simulink library "TMCA_lib"  (Simulink 7.5)
settings: Solver=ode45  StartTime=0.0  StopTime=10.0  RelTol=1e-3
values from neighbouring files (symbols this model uses):
  pTMCA_A_BatCurrHi_C = Simulink.Parameter    [TMCA_par.m]
  pTMCA_A_BatCurrLo_C = Simulink.Parameter    [TMCA_par.m]
  pTMCA_bool_ACPtcConfig_C = Simulink.Parameter    [TMCA_par.m]
  pTMCA_bool_BatCoolACReqCtrl_C = Simulink.Parameter    [TMCA_par.m]
  pTMCA_bool_BatCoolACReqEnbl_C = Simulink.Parameter    [TMCA_par.m]
  pTMCA_bool_BatCoolEnbl_C = Simulink.Parameter    [TMCA_par.m]
  pTMCA_bool_BatHeatEnbl_C = Simulink.Parameter    [TMCA_par.m]
  pTMCA_bool_ChrgrValveCtrl_C = Simulink.Parameter    [TMCA_par.m]
  pTMCA_bool_ChrgrValveEnbl_C = Simulink.Parameter    [TMCA_par.m]
  pTMCA_bool_FanCtrlEnbl = Simulink.Parameter    [TMCA_par.m]
  pTMCA_bool_FanCtrlSwitch = Simulink.Parameter    [TMCA_par.m]
  pTMCA_bool_Mot1PmpEnbl_C = Simulink.Parameter    [TMCA_par.m]
  pTMCA_bool_Mot2PmpEnbl_C = Simulink.Parameter    [TMCA_par.m]
  pTMCA_bool_MotValveCtrl_C = Simulink.Parameter    [TMCA_par.m]
  pTMCA_bool_MotValveEnbl_C = Simulink.Parameter    [TMCA_par.m]
  pTMCA_bool_TMCoolEnbl_C = Simulink.Parameter    [TMCA_par.m]
  pTMCA_bool_WtrPmpCoolEnbl_C = Simulink.Parameter    [TMCA_par.m]
  pTMCA_bool_WtrPmpHeatEnbl_C = Simulink.Parameter    [TMCA_par.m]
  pTMCA_cnt_ACHeatTime_CUR = Simulink.Parameter    [TMCA_par.m]
  pTMCA_cnt_DCTempTime_CUR = Simulink.Parameter    [TMCA_par.m]
  pTMCA_cnt_TimeDwnLim_C = Simulink.Parameter    [TMCA_par.m]
  pTMCA_cnt_TimeUpLim_C = Simulink.Parameter    [TMCA_par.m]
  pTMCA_degC_AmbHiTempDisply_C = Simulink.Parameter    [TMCA_par.m]
  pTMCA_degC_BatCoolAmbHiTemp_C = Simulink.Parameter    [TMCA_par.m]
  pTMCA_degC_BatCoolAmbLoTemp_C = Simulink.Parameter    [TMCA_par.m]
  pTMCA_degC_BatCoolHiTemp_C = Simulink.Parameter    [TMCA_par.m]
  pTMCA_degC_BatCoolLoTemp_C = Simulink.Parameter    [TMCA_par.m]
  pTMCA_degC_BatHiTempDisply_C = Simulink.Parameter    [TMCA_par.m]
  pTMCA_degC_BatMaxT_CUR = Simulink.Parameter    [TMCA_par.m]
  pTMCA_degC_BatMaxTHiThd_C = Simulink.Parameter    [TMCA_par.m]
  pTMCA_degC_BatMaxTLoThd_C = Simulink.Parameter    [TMCA_par.m]
  pTMCA_degC_ChrgrHiTThd_C = Simulink.Parameter    [TMCA_par.m]
  pTMCA_degC_ChrgrLoTThd_C = Simulink.Parameter    [TMCA_par.m]
  pTMCA_degC_ChrgrTThd_CUR = Simulink.Parameter    [TMCA_par.m]
  pTMCA_degC_DcDcHiTThd_C = Simulink.Parameter    [TMCA_par.m]
  pTMCA_degC_DcDcLoTThd_C = Simulink.Parameter    [TMCA_par.m]
  pTMCA_degC_DcDcTThd_CUR = Simulink.Parameter    [TMCA_par.m]
  pTMCA_degC_MotWtrHiTThd_C = Simulink.Parameter    [TMCA_par.m]
  pTMCA_degC_MotWtrLoTThd_C = Simulink.Parameter    [TMCA_par.m]
  pTMCA_degC_MotWtrMaxTThd_C = Simulink.Parameter    [TMCA_par.m]
  pTMCA_degC_MotWtrMinTThd_C = Simulink.Parameter    [TMCA_par.m]
  pTMCA_pct_ACHeatPTCPWM_CUR = Simulink.Parameter    [TMCA_par.m]
  pTMCA_pct_BatWtrPmpPWM_CUR = Simulink.Parameter    [TMCA_par.m]
  pTMCA_pct_ChrgrWtrPmpPWM_CUR = Simulink.Parameter    [TMCA_par.m]
  pTMCA_pct_DcDcWtrPmpPWM_CUR = Simulink.Parameter    [TMCA_par.m]
  pTMCA_pct_DCHeatPTCPWM_CUR = Simulink.Parameter    [TMCA_par.m]
  pTMCA_pct_HeatPTCCtrl_C = Simulink.Parameter    [TMCA_par.m]
  pTMCA_pct_HeatPTCEnbl_C = Simulink.Parameter    [TMCA_par.m]
  pTMCA_pct_HeatrOffVal_C = Simulink.Parameter    [TMCA_par.m]
  pTMCA_pct_Mot1PmpPWMCtrl_C = Simulink.Parameter    [TMCA_par.m]
  pTMCA_pct_Mot2PmpPWMCtrl_C = Simulink.Parameter    [TMCA_par.m]
  pTMCA_pct_MotWtrPmpMaxSpd_C = Simulink.Parameter    [TMCA_par.m]
  pTMCA_pct_MotWtrPmpMinSpd_C = Simulink.Parameter    [TMCA_par.m]
  pTMCA_pct_MotWtrPmpNormSpd_C = Simulink.Parameter    [TMCA_par.m]
  pTMCA_pct_MotWtrPmpZeroSpd_C = Simulink.Parameter    [TMCA_par.m]
  pTMCA_pct_WtrPmpCoolCtrl_C = Simulink.Parameter    [TMCA_par.m]
  pTMCA_pct_WtrPmpHeatCtrl_C = Simulink.Parameter    [TMCA_par.m]
  pTMCA_s_ACDisChrgTimout_C = Simulink.Parameter    [TMCA_par.m]
  pTMCA_s_TFilSampleTi_C = Simulink.Parameter    [TMCA_par.m]
  pTMCA_st_AirCdnOn_C = Simulink.Parameter    [TMCA_par.m]
undefined symbols (not defined in the file or in its folder): AirCdnFanReqTyp, ChrgActStsTyp, MCUCoolReqTyp, p_bool_False_M, p_bool_True_M, PUDCoorrStsTyp
libraries: BaseOperationLib_Browser x197, PES_CZ_FAW x3, simulink x1
(part 1 of 2)
settings Model: Creator=wuaibin  LastModifiedBy=wuaibin

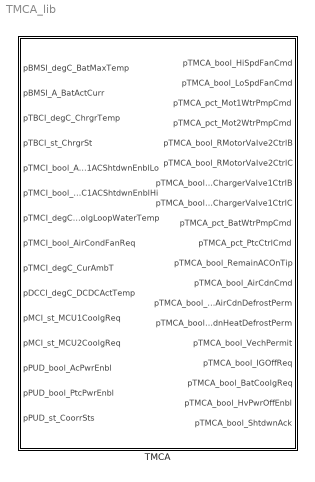
== system TMCA_lib ==
  TMCA : Subsystem  TreatAsAtomicUnit=on

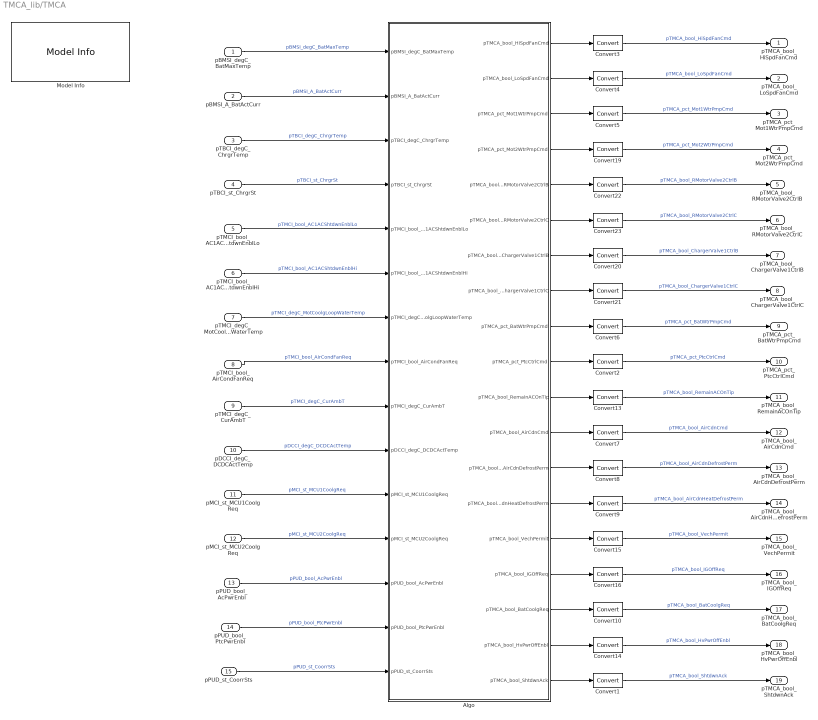
== system TMCA_lib/TMCA ==
  pBMSI_degC_BatMaxTemp : Inport  OutDataType=fixdt(1, 16)  OutScaling=2^0
  pBMSI_A_BatActCurr : Inport  Port=2  OutDataType=fixdt(1, 16)  OutScaling=2^0
  pTBCI_degC_ChrgrTemp : Inport  Port=3  OutDataType=fixdt(1, 16)  OutScaling=2^0
  pTBCI_st_ChrgrSt : Inport  Port=4  OutDataType=fixdt(1, 16)  OutScaling=2^0
  pTMCI_bool_AC1ACShtdwnEnblLo : Inport  Port=5  OutDataType=fixdt(1, 16)  OutScaling=2^0
  pTMCI_bool_AC1ACShtdwnEnblHi : Inport  Port=6  OutDataType=fixdt(1, 16)  OutScaling=2^0
  pTMCI_degC_MotCoolgLoopWaterTemp : Inport  Port=7  OutDataType=fixdt(1, 16)  OutScaling=2^0
  pTMCI_bool_AirCondFanReq : Inport  Port=8  OutDataType=fixdt(1, 16)  OutScaling=2^0
  pTMCI_degC_CurAmbT : Inport  Port=9  OutDataType=fixdt(1, 16)  OutScaling=2^0
  pDCCI_degC_DCDCActTemp : Inport  Port=10  OutDataType=fixdt(1, 16)  OutScaling=2^0
  pMCI_st_MCU1CoolgReq : Inport  Port=11  OutDataType=fixdt(1, 16)  OutScaling=2^0
  pMCI_st_MCU2CoolgReq : Inport  Port=12  OutDataType=fixdt(1, 16)  OutScaling=2^0
  pPUD_bool_AcPwrEnbl : Inport  Port=13
  pPUD_bool_PtcPwrEnbl : Inport  Port=14  OutDataType=fixdt(1, 16)  OutScaling=2^0
  pPUD_st_CoorrSts : Inport  Port=15
  Algo : Subsystem
  Convert{1..10,13..16,19..23} (19 alike) : DataTypeConversion  OutDataType=fixdt(1, 16)  OutScaling=2^0
  Model Info : simulink/Model-Wide Utilities/Model Info  SystemSampleTime=-1  InitialBlockCM=None  BlockCM=None  Frame=on  DisplayStringWithTags=Model Info\nCreated: %<Created>\nCreator: zhangqiang  HorizontalTextAlignment=Center  LeftAlignmentValue=0.5  SourceBlockDiagram=HQEV_HCU  TagMaxNumber=20
  pTMCA_bool_HiSpdFanCmd : Outport  OutDataType=fixdt(1, 16)  OutScaling=2^0
  pTMCA_bool_LoSpdFanCmd : Outport  Port=2  OutDataType=fixdt(1, 16)  OutScaling=2^0
  pTMCA_pct_Mot1WtrPmpCmd : Outport  Port=3  OutDataType=fixdt(1, 16)  OutScaling=2^0
  pTMCA_pct_Mot2WtrPmpCmd : Outport  Port=4  OutDataType=fixdt(1, 16)  OutScaling=2^0
  pTMCA_bool_RMotorValve2CtrlB : Outport  Port=5
  pTMCA_bool_RMotorValve2CtrlC : Outport  Port=6
  pTMCA_bool_ChargerValve1CtrlB : Outport  Port=7
  pTMCA_bool_ChargerValve1CtrlC : Outport  Port=8
  pTMCA_pct_BatWtrPmpCmd : Outport  Port=9  OutDataType=fixdt(1, 16)  OutScaling=2^0
  pTMCA_pct_PtcCtrlCmd : Outport  Port=10  OutDataType=fixdt(1, 16)  OutScaling=2^0
  pTMCA_bool_RemainACOnTip : Outport  Port=11  OutDataType=fixdt(1, 16)  OutScaling=2^0
  pTMCA_bool_AirCdnCmd : Outport  Port=12  OutDataType=fixdt(1, 16)  OutScaling=2^0
  pTMCA_bool_AirCdnDefrostPerm : Outport  Port=13  OutDataType=fixdt(1, 16)  OutScaling=2^0
  pTMCA_bool_AirCdnHeatDefrostPerm : Outport  Port=14  OutDataType=fixdt(1, 16)  OutScaling=2^0
  pTMCA_bool_VechPermit : Outport  Port=15  OutDataType=fixdt(1, 16)  OutScaling=2^0
  pTMCA_bool_IGOffReq : Outport  Port=16  OutDataType=fixdt(1, 16)  OutScaling=2^0
  pTMCA_bool_BatCoolgReq : Outport  Port=17  OutDataType=fixdt(1, 16)  OutScaling=2^0
  pTMCA_bool_HvPwrOffEnbl : Outport  Port=18  OutDataType=fixdt(1, 16)  OutScaling=2^0
  pTMCA_bool_ShtdwnAck : Outport  Port=19  OutDataType=fixdt(1, 16)  OutScaling=2^0
  wires:
  Convert2/1 -> pTMCA_pct_PtcCtrlCmd/1  "pTMCA_pct_PtcCtrlCmd"
  Convert5/1 -> pTMCA_pct_Mot1WtrPmpCmd/1  "pTMCA_pct_Mot1WtrPmpCmd"
  Convert6/1 -> pTMCA_pct_BatWtrPmpCmd/1  "pTMCA_pct_BatWtrPmpCmd"
  Convert10/1 -> pTMCA_bool_BatCoolgReq/1  "pTMCA_bool_BatCoolgReq"
  Convert19/1 -> pTMCA_pct_Mot2WtrPmpCmd/1  "pTMCA_pct_Mot2WtrPmpCmd"
  Convert13/1 -> pTMCA_bool_RemainACOnTip/1  "pTMCA_bool_RemainACOnTip"
  pPUD_st_CoorrSts/1 -> Algo/15(pPUD_st_CoorrSts)  "pPUD_st_CoorrSts"
  pPUD_bool_PtcPwrEnbl/1 -> Algo/14(pPUD_bool_PtcPwrEnbl)  "pPUD_bool_PtcPwrEnbl"
  pTMCI_degC_MotCoolgLoopWaterTemp/1 -> Algo/7(pTMCI_degC_MotCoolgLoopWaterTemp)  "pTMCI_degC_MotCoolgLoopWaterTemp"
  pTMCI_bool_AirCondFanReq/1 -> Algo/8(pTMCI_bool_AirCondFanReq)  "pTMCI_bool_AirCondFanReq"
  pTBCI_st_ChrgrSt/1 -> Algo/4(pTBCI_st_ChrgrSt)  "pTBCI_st_ChrgrSt"
  pTBCI_degC_ChrgrTemp/1 -> Algo/3(pTBCI_degC_ChrgrTemp)  "pTBCI_degC_ChrgrTemp"
  pDCCI_degC_DCDCActTemp/1 -> Algo/10(pDCCI_degC_DCDCActTemp)  "pDCCI_degC_DCDCActTemp"
  pMCI_st_MCU1CoolgReq/1 -> Algo/11(pMCI_st_MCU1CoolgReq)  "pMCI_st_MCU1CoolgReq"
  pMCI_st_MCU2CoolgReq/1 -> Algo/12(pMCI_st_MCU2CoolgReq)  "pMCI_st_MCU2CoolgReq"
  pBMSI_degC_BatMaxTemp/1 -> Algo/1(pBMSI_degC_BatMaxTemp)  "pBMSI_degC_BatMaxTemp"
  pTMCI_degC_CurAmbT/1 -> Algo/9(pTMCI_degC_CurAmbT)  "pTMCI_degC_CurAmbT"
  pPUD_bool_AcPwrEnbl/1 -> Algo/13(pPUD_bool_AcPwrEnbl)  "pPUD_bool_AcPwrEnbl"
  pBMSI_A_BatActCurr/1 -> Algo/2(pBMSI_A_BatActCurr)  "pBMSI_A_BatActCurr"
  pTMCI_bool_AC1ACShtdwnEnblLo/1 -> Algo/5(pTMCI_bool_AC1ACShtdwnEnblLo)  "pTMCI_bool_AC1ACShtdwnEnblLo"
  pTMCI_bool_AC1ACShtdwnEnblHi/1 -> Algo/6(pTMCI_bool_AC1ACShtdwnEnblHi)  "pTMCI_bool_AC1ACShtdwnEnblHi"
  Algo/1(pTMCA_bool_HiSpdFanCmd) -> Convert3/1
  Algo/2(pTMCA_bool_LoSpdFanCmd) -> Convert4/1
  Algo/3(pTMCA_pct_Mot1WtrPmpCmd) -> Convert5/1
  Algo/4(pTMCA_pct_Mot2WtrPmpCmd) -> Convert19/1
  Algo/5(pTMCA_bool_RMotorValve2CtrlB) -> Convert22/1
  Algo/6(pTMCA_bool_RMotorValve2CtrlC) -> Convert23/1
  Algo/7(pTMCA_bool_ChargerValve1CtrlB) -> Convert20/1
  Algo/8(pTMCA_bool_ChargerValve1CtrlC) -> Convert21/1
  Algo/9(pTMCA_pct_BatWtrPmpCmd) -> Convert6/1
  Algo/10(pTMCA_pct_PtcCtrlCmd) -> Convert2/1
  Algo/11(pTMCA_bool_RemainACOnTip) -> Convert13/1
  Algo/12(pTMCA_bool_AirCdnCmd) -> Convert7/1
  Algo/13(pTMCA_bool_AirCdnDefrostPerm) -> Convert8/1
  Algo/14(pTMCA_bool_AirCdnHeatDefrostPerm) -> Convert9/1
  Algo/15(pTMCA_bool_VechPermit) -> Convert15/1
  Algo/16(pTMCA_bool_IGOffReq) -> Convert16/1
  Algo/17(pTMCA_bool_BatCoolgReq) -> Convert10/1
  Algo/18(pTMCA_bool_HvPwrOffEnbl) -> Convert14/1
  Convert3/1 -> pTMCA_bool_HiSpdFanCmd/1  "pTMCA_bool_HiSpdFanCmd"
  Convert4/1 -> pTMCA_bool_LoSpdFanCmd/1  "pTMCA_bool_LoSpdFanCmd"
  Convert22/1 -> pTMCA_bool_RMotorValve2CtrlB/1  "pTMCA_bool_RMotorValve2CtrlB"
  Convert23/1 -> pTMCA_bool_RMotorValve2CtrlC/1  "pTMCA_bool_RMotorValve2CtrlC"
  Convert20/1 -> pTMCA_bool_ChargerValve1CtrlB/1  "pTMCA_bool_ChargerValve1CtrlB"
  Convert21/1 -> pTMCA_bool_ChargerValve1CtrlC/1  "pTMCA_bool_ChargerValve1CtrlC"
  Convert7/1 -> pTMCA_bool_AirCdnCmd/1  "pTMCA_bool_AirCdnCmd"
  Convert8/1 -> pTMCA_bool_AirCdnDefrostPerm/1  "pTMCA_bool_AirCdnDefrostPerm"
  Convert9/1 -> pTMCA_bool_AirCdnHeatDefrostPerm/1  "pTMCA_bool_AirCdnHeatDefrostPerm"
  Convert15/1 -> pTMCA_bool_VechPermit/1  "pTMCA_bool_VechPermit"
  Convert16/1 -> pTMCA_bool_IGOffReq/1  "pTMCA_bool_IGOffReq"
  Convert1/1 -> pTMCA_bool_ShtdwnAck/1  "pTMCA_bool_ShtdwnAck"
  Convert14/1 -> pTMCA_bool_HvPwrOffEnbl/1  "pTMCA_bool_HvPwrOffEnbl"
  Algo/19(pTMCA_bool_ShtdwnAck) -> Convert1/1

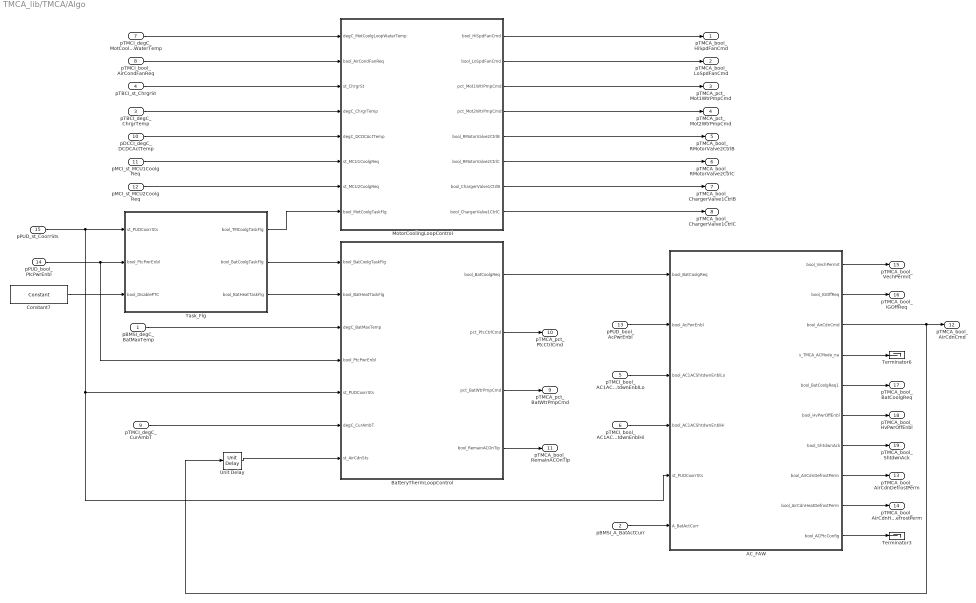
== system TMCA_lib/TMCA/Algo ==
  pBMSI_degC_BatMaxTemp : Inport  OutDataType=fixdt(1, 16)  OutScaling=2^0
  pBMSI_A_BatActCurr : Inport  Port=2  OutDataType=fixdt(1, 16)  OutScaling=2^0
  pTBCI_degC_ChrgrTemp : Inport  Port=3  OutDataType=fixdt(1, 16)  OutScaling=2^0
  pTBCI_st_ChrgrSt : Inport  Port=4  OutDataType=fixdt(1, 16)  OutScaling=2^0
  pTMCI_bool_AC1ACShtdwnEnblLo : Inport  Port=5  OutDataType=fixdt(1, 16)  OutScaling=2^0
  pTMCI_bool_AC1ACShtdwnEnblHi : Inport  Port=6  OutDataType=fixdt(1, 16)  OutScaling=2^0
  pTMCI_degC_MotCoolgLoopWaterTemp : Inport  Port=7  OutDataType=fixdt(1, 16)  OutScaling=2^0
  pTMCI_bool_AirCondFanReq : Inport  Port=8  OutDataType=fixdt(1, 16)  OutScaling=2^0
  pTMCI_degC_CurAmbT : Inport  Port=9  OutDataType=fixdt(1, 16)  OutScaling=2^0
  pDCCI_degC_DCDCActTemp : Inport  Port=10  OutDataType=fixdt(1, 16)  OutScaling=2^0
  pMCI_st_MCU1CoolgReq : Inport  Port=11  OutDataType=fixdt(1, 16)  OutScaling=2^0
  pMCI_st_MCU2CoolgReq : Inport  Port=12  OutDataType=fixdt(1, 16)  OutScaling=2^0
  pPUD_bool_AcPwrEnbl : Inport  Port=13  OutDataType=fixdt(1, 16)  OutScaling=2^0
  pPUD_bool_PtcPwrEnbl : Inport  Port=14
  pPUD_st_CoorrSts : Inport  Port=15  OutDataType=fixdt(1, 16)  OutScaling=2^0
  AC_FAW : Subsystem
  BatteryThermLoopControl : Subsystem
  Constant7 : BaseOperationLib_Browser/Sources&Sinks/Constant  Value=p_bool_False_M  OutMin=[]  OutMax=[]  OutDataType=fixdt(1, 16)  ConRadixGroup=Use specified scaling  OutScaling=2^0  OutDataTypeStr=Inherit: Inherit from 'Constant value'
  MotorCoolingLoopControl : Subsystem
  Task_Flg : Subsystem
  Terminator3 : Terminator
  Terminator6 : Terminator
  Unit Delay : BaseOperationLib_Browser/Discrete Unchanged /Unit Delay  X0=0  SampleTime=-1
  pTMCA_bool_HiSpdFanCmd : Outport  OutDataType=fixdt(1, 16)  OutScaling=2^0
  pTMCA_bool_LoSpdFanCmd : Outport  Port=2  OutDataType=fixdt(1, 16)  OutScaling=2^0
  pTMCA_pct_Mot1WtrPmpCmd : Outport  Port=3  OutDataType=fixdt(1, 16)  OutScaling=2^0
  pTMCA_pct_Mot2WtrPmpCmd : Outport  Port=4  PortDimensions=1  OutDataType=fixdt(1, 16)  OutScaling=2^0
  pTMCA_bool_RMotorValve2CtrlB : Outport  Port=5
  pTMCA_bool_RMotorValve2CtrlC : Outport  Port=6
  pTMCA_bool_ChargerValve1CtrlB : Outport  Port=7
  pTMCA_bool_ChargerValve1CtrlC : Outport  Port=8
  pTMCA_pct_BatWtrPmpCmd : Outport  Port=9  OutDataType=fixdt(1, 16)  OutScaling=2^0
  pTMCA_pct_PtcCtrlCmd : Outport  Port=10  OutDataType=fixdt(1, 16)  OutScaling=2^0
  pTMCA_bool_RemainACOnTip : Outport  Port=11  OutDataType=fixdt(1, 16)  OutScaling=2^0
  pTMCA_bool_AirCdnCmd : Outport  Port=12  OutDataType=fixdt(1, 16)  OutScaling=2^0
  pTMCA_bool_AirCdnDefrostPerm : Outport  Port=13  OutDataType=fixdt(1, 16)  OutScaling=2^0
  pTMCA_bool_AirCdnHeatDefrostPerm : Outport  Port=14  OutDataType=fixdt(1, 16)  OutScaling=2^0
  pTMCA_bool_VechPermit : Outport  Port=15  OutDataType=fixdt(1, 16)  OutScaling=2^0
  pTMCA_bool_IGOffReq : Outport  Port=16  OutDataType=fixdt(1, 16)  OutScaling=2^0
  pTMCA_bool_BatCoolgReq : Outport  Port=17  OutDataType=fixdt(1, 16)  OutScaling=2^0
  pTMCA_bool_HvPwrOffEnbl : Outport  Port=18  OutDataType=fixdt(1, 16)  OutScaling=2^0
  pTMCA_bool_ShtdwnAck : Outport  Port=19  OutDataType=fixdt(1, 16)  OutScaling=2^0
  wires:
  AC_FAW/3(bool_AirCdnCmd) -> pTMCA_bool_AirCdnCmd/1, Unit Delay/1
  Unit Delay/1 -> BatteryThermLoopControl/7(st_AirCdnSts)
  pTMCI_bool_AC1ACShtdwnEnblLo/1 -> AC_FAW/3(bool_AC1ACShtdwnEnblLo)
  AC_FAW/5(bool_BatCoolgReq1) -> pTMCA_bool_BatCoolgReq/1
  AC_FAW/4(s_TMCA_ACMode_na) -> Terminator6/1
  AC_FAW/8(bool_AirCdnDefrostPerm) -> pTMCA_bool_AirCdnDefrostPerm/1
  AC_FAW/9(bool_AirCdnHeatDefrostPerm) -> pTMCA_bool_AirCdnHeatDefrostPerm/1
  pTMCI_degC_MotCoolgLoopWaterTemp/1 -> MotorCoolingLoopControl/1(degC_MotCoolgLoopWaterTemp)
  pTMCI_bool_AirCondFanReq/1 -> MotorCoolingLoopControl/2(bool_AirCondFanReq)
  MotorCoolingLoopControl/2(bool_LoSpdFanCmd) -> pTMCA_bool_LoSpdFanCmd/1
  MotorCoolingLoopControl/1(bool_HiSpdFanCmd) -> pTMCA_bool_HiSpdFanCmd/1
  AC_FAW/10(bool_ACPtcConfig) -> Terminator3/1
  AC_FAW/1(bool_VechPermit) -> pTMCA_bool_VechPermit/1
  AC_FAW/2(bool_IGOffReq) -> pTMCA_bool_IGOffReq/1
  pTMCI_degC_CurAmbT/1 -> BatteryThermLoopControl/6(degC_CurAmbT)
  pTBCI_degC_ChrgrTemp/1 -> MotorCoolingLoopControl/4(degC_ChrgrTemp)
  pDCCI_degC_DCDCActTemp/1 -> MotorCoolingLoopControl/5(degC_DCDCActTemp)
  pMCI_st_MCU1CoolgReq/1 -> MotorCoolingLoopControl/6(st_MCU1CoolgReq)
  pMCI_st_MCU2CoolgReq/1 -> MotorCoolingLoopControl/7(st_MCU2CoolgReq)
  MotorCoolingLoopControl/3(pct_Mot1WtrPmpCmd) -> pTMCA_pct_Mot1WtrPmpCmd/1
  pBMSI_degC_BatMaxTemp/1 -> BatteryThermLoopControl/3(degC_BatMaxTemp)
  BatteryThermLoopControl/3(pct_BatWtrPmpCmd) -> pTMCA_pct_BatWtrPmpCmd/1
  BatteryThermLoopControl/1(bool_BatCoolgReq) -> AC_FAW/1(bool_BatCoolgReq)
  pPUD_bool_AcPwrEnbl/1 -> AC_FAW/2(bool_AcPwrEnbl)
  MotorCoolingLoopControl/4(pct_Mot2WtrPmpCmd) -> pTMCA_pct_Mot2WtrPmpCmd/1
  pTBCI_st_ChrgrSt/1 -> MotorCoolingLoopControl/3(st_ChrgrSt)
  MotorCoolingLoopControl/7(bool_ChargerValve1CtrlB) -> pTMCA_bool_ChargerValve1CtrlB/1
  MotorCoolingLoopControl/8(bool_ChargerValve1CtrlC) -> pTMCA_bool_ChargerValve1CtrlC/1
  MotorCoolingLoopControl/5(bool_RMotorValve2CtrlB) -> pTMCA_bool_RMotorValve2CtrlB/1
  MotorCoolingLoopControl/6(bool_RMotorValve2CtrlC) -> pTMCA_bool_RMotorValve2CtrlC/1
  BatteryThermLoopControl/4(bool_RemainACOnTip) -> pTMCA_bool_RemainACOnTip/1
  AC_FAW/6(bool_HvPwrOffEnbl) -> pTMCA_bool_HvPwrOffEnbl/1
  pPUD_bool_PtcPwrEnbl/1 -> BatteryThermLoopControl/4(bool_PtcPwrEnbl), Task_Flg/2(bool_PtcPwrEnbl)
  Constant7/1 -> Task_Flg/3(bool_DisablePTC)
  AC_FAW/7(bool_ShtdwnAck) -> pTMCA_bool_ShtdwnAck/1
  BatteryThermLoopControl/2(pct_PtcCtrlCmd) -> pTMCA_pct_PtcCtrlCmd/1
  Task_Flg/1(bool_TMCoolgTaskFlg) -> MotorCoolingLoopControl/8(bool_MotCoolgTaskFlg)
  Task_Flg/2(bool_BatCoolgTaskFlg) -> BatteryThermLoopControl/1(bool_BatCoolgTaskFlg)
  Task_Flg/3(bool_BatHeatTaskFlg) -> BatteryThermLoopControl/2(bool_BatHeatTaskFlg)
  pPUD_st_CoorrSts/1 -> Task_Flg/1(st_PUDCoorrSts), BatteryThermLoopControl/5(st_PUDCoorrSts), AC_FAW/5(st_PUDCoorrSts)
  pTMCI_bool_AC1ACShtdwnEnblHi/1 -> AC_FAW/4(bool_AC1ACShtdwnEnblHi)
  pBMSI_A_BatActCurr/1 -> AC_FAW/6(A_BatActCurr)

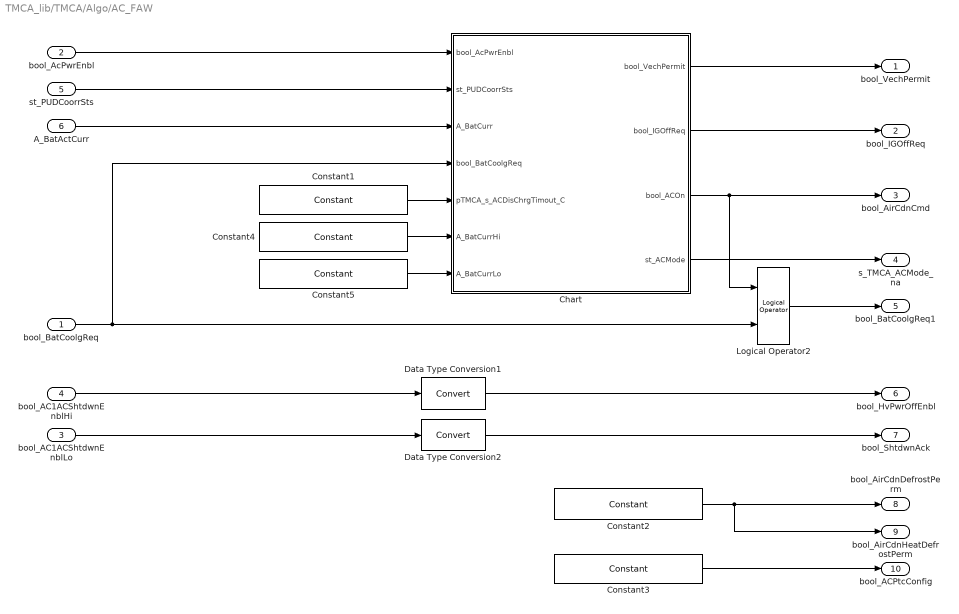
== system TMCA_lib/TMCA/Algo/AC_FAW ==
  bool_BatCoolgReq : Inport  OutDataType=fixdt(1, 16)  OutScaling=2^0
  bool_AcPwrEnbl : Inport  Port=2  OutDataType=fixdt(1, 16)  OutScaling=2^0
  bool_AC1ACShtdwnEnblLo : Inport  Port=3  OutDataType=fixdt(1, 16)  OutScaling=2^0
  bool_AC1ACShtdwnEnblHi : Inport  Port=4  OutDataType=fixdt(1, 16)  OutScaling=2^0
  st_PUDCoorrSts : Inport  Port=5  OutDataType=fixdt(1, 16)  OutScaling=2^0
  A_BatActCurr : Inport  Port=6  OutDataType=fixdt(1, 16)  OutScaling=2^0
  Chart : Stateflow chart  TreatAsAtomicUnit=on
  Constant1 : BaseOperationLib_Browser/Sources&Sinks/Constant  Value=pTMCA_s_ACDisChrgTimout_C  OutMin=[]  OutMax=[]  OutDataType=fixdt(1, 16)  ConRadixGroup=Use specified scaling  OutScaling=2^0  OutDataTypeStr=Inherit: Inherit from 'Constant value'
  Constant2 : BaseOperationLib_Browser/Sources&Sinks/Constant  Value=p_bool_False_M  OutMin=[]  OutMax=[]  OutDataType=fixdt(1, 16)  ConRadixGroup=Use specified scaling  OutScaling=2^0  OutDataTypeStr=Inherit: Inherit from 'Constant value'
  Constant3 : BaseOperationLib_Browser/Sources&Sinks/Constant  Value=pTMCA_bool_ACPtcConfig_C  OutMin=[]  OutMax=[]  OutDataType=fixdt(1, 16)  ConRadixGroup=Use specified scaling  OutScaling=2^0  OutDataTypeStr=Inherit: Inherit from 'Constant value'
  Constant4 : BaseOperationLib_Browser/Sources&Sinks/Constant  Value=pTMCA_A_BatCurrHi_C  OutMin=[]  OutMax=[]  OutDataType=fixdt(1, 16)  ConRadixGroup=Use specified scaling  OutScaling=2^0  OutDataTypeStr=Inherit: Inherit from 'Constant value'
  Constant5 : BaseOperationLib_Browser/Sources&Sinks/Constant  Value=pTMCA_A_BatCurrLo_C  OutMin=[]  OutMax=[]  OutDataType=fixdt(1, 16)  ConRadixGroup=Use specified scaling  OutScaling=2^0  OutDataTypeStr=Inherit: Inherit from 'Constant value'
  Data Type Conversion1 : DataTypeConversion  OutDataType=fixdt(1, 16)  OutScaling=2^0
  Data Type Conversion2 : DataTypeConversion  OutDataType=fixdt(1, 16)  OutScaling=2^0
  Logical Operator2 : BaseOperationLib_Browser/Logic Operations Changed/Logical Operator  Operator=AND  Inputs=2  AllPortsSameDT=on  OutDataTypeMode=Specify via dialog  LogicDataType=PDT_Bool  OutDataTypeStr=PDT_Bool
  bool_VechPermit : Outport  OutDataType=fixdt(1, 16)  OutScaling=2^0
  bool_IGOffReq : Outport  Port=2  OutDataType=fixdt(1, 16)  OutScaling=2^0
  bool_AirCdnCmd : Outport  Port=3  OutDataType=fixdt(1, 16)  OutScaling=2^0
  s_TMCA_ACMode_na : Outport  Port=4  PortDimensions=1  OutDataType=fixdt(1, 16)  OutScaling=2^0
  bool_BatCoolgReq1 : Outport  Port=5  OutDataType=fixdt(1, 16)  OutScaling=2^0
  bool_HvPwrOffEnbl : Outport  Port=6  PortDimensions=1  OutDataType=fixdt(1, 16)  OutScaling=2^0
  bool_ShtdwnAck : Outport  Port=7  OutDataType=fixdt(1, 16)  OutScaling=2^0
  bool_AirCdnDefrostPerm : Outport  Port=8  OutDataType=fixdt(1, 16)  OutScaling=2^0
  bool_AirCdnHeatDefrostPerm : Outport  Port=9  OutDataType=fixdt(1, 16)  OutScaling=2^0
  bool_ACPtcConfig : Outport  Port=10  OutDataType=fixdt(1, 16)  OutScaling=2^0
  wires:
  st_PUDCoorrSts/1 -> Chart/2(st_PUDCoorrSts)
  Logical Operator2/1 -> bool_BatCoolgReq1/1
  bool_BatCoolgReq/1 -> Logical Operator2/2, Chart/4(bool_BatCoolgReq)
  Chart/4(st_ACMode) -> s_TMCA_ACMode_na/1
  Chart/3(bool_ACOn) -> bool_AirCdnCmd/1, Logical Operator2/1
  Chart/2(bool_IGOffReq) -> bool_IGOffReq/1
  bool_AcPwrEnbl/1 -> Chart/1(bool_AcPwrEnbl)
  Chart/1(bool_VechPermit) -> bool_VechPermit/1
  Constant2/1 -> bool_AirCdnDefrostPerm/1, bool_AirCdnHeatDefrostPerm/1
  Constant3/1 -> bool_ACPtcConfig/1
  Data Type Conversion1/1 -> bool_HvPwrOffEnbl/1
  bool_AC1ACShtdwnEnblHi/1 -> Data Type Conversion1/1
  bool_AC1ACShtdwnEnblLo/1 -> Data Type Conversion2/1
  Data Type Conversion2/1 -> bool_ShtdwnAck/1
  A_BatActCurr/1 -> Chart/3(A_BatCurr)
  Constant1/1 -> Chart/5(pTMCA_s_ACDisChrgTimout_C)
  Constant4/1 -> Chart/6(A_BatCurrHi)
  Constant5/1 -> Chart/7(A_BatCurrLo)

== system TMCA_lib/TMCA/Algo/BatteryThermLoopControl ==
  bool_BatCoolgTaskFlg : Inport  OutDataType=fixdt(1, 16)  OutScaling=2^0
  bool_BatHeatTaskFlg : Inport  Port=2  OutDataType=fixdt(1, 16)  OutScaling=2^0
  degC_BatMaxTemp : Inport  Port=3  OutDataType=fixdt(1, 16)  OutScaling=2^0
  bool_PtcPwrEnbl : Inport  Port=4  OutDataType=fixdt(1, 16)  OutScaling=2^0
  st_PUDCoorrSts : Inport  Port=5  OutDataType=fixdt(1, 16)  OutScaling=2^0
  degC_CurAmbT : Inport  Port=6  OutDataType=fixdt(1, 16)  OutScaling=2^0
  st_AirCdnSts : Inport  Port=7  OutDataType=fixdt(1, 16)  OutScaling=2^0
  BatCoolingCtrl : Subsystem
  BatHeatingCtrl : Subsystem
  BatWaterPmpCtrl : Subsystem
  bool_BatCoolgReq : Outport  OutDataType=fixdt(1, 16)  OutScaling=2^0
  pct_PtcCtrlCmd : Outport  Port=2  OutDataType=fixdt(1, 16)  OutScaling=2^0
  pct_BatWtrPmpCmd : Outport  Port=3  OutDataType=fixdt(1, 16)  OutScaling=2^0
  bool_RemainACOnTip : Outport  Port=4  OutDataType=fixdt(1, 16)  OutScaling=2^0
  wires:
  bool_PtcPwrEnbl/1 -> BatHeatingCtrl/1(bool_PtcPwrEnbl)
  st_AirCdnSts/1 -> BatCoolingCtrl/3(st_AirCdnSts)
  degC_BatMaxTemp/1 -> BatCoolingCtrl/1(degC_BatMaxTemp), BatWaterPmpCtrl/3(degC_BatMaxTemp)
  BatHeatingCtrl/1(pct_PtcCtrlCmd) -> BatWaterPmpCtrl/2(pct_PtcCtrlCmd), pct_PtcCtrlCmd/1
  BatCoolingCtrl/1(bool_BatCoolgReq) -> BatWaterPmpCtrl/1(bool_BatCoolgReq), bool_BatCoolgReq/1
  BatWaterPmpCtrl/1(pct_BatWtrPmpCmd) -> pct_BatWtrPmpCmd/1
  BatCoolingCtrl/2(bool_RemainACOnTip) -> bool_RemainACOnTip/1
  degC_CurAmbT/1 -> BatCoolingCtrl/2(degC_CurAmbT)
  bool_BatCoolgTaskFlg/1 -> BatWaterPmpCtrl/4(bool_BatCoolgTaskFlg), BatCoolingCtrl/4(bool_BatCoolgTaskFlg)
  bool_BatHeatTaskFlg/1 -> BatHeatingCtrl/3(bool_BatHeatTaskFlg), BatWaterPmpCtrl/5(bool_BatHeatTaskFlg)
  st_PUDCoorrSts/1 -> BatHeatingCtrl/2(st_PUDCoorrSts)

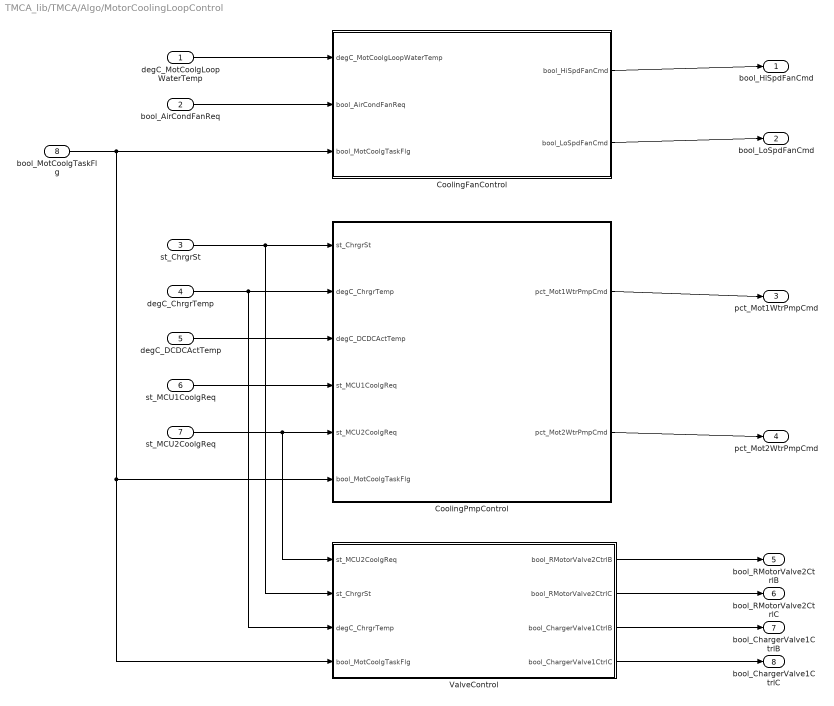
== system TMCA_lib/TMCA/Algo/MotorCoolingLoopControl ==
  degC_MotCoolgLoopWaterTemp : Inport  OutDataType=fixdt(1, 16)  OutScaling=2^0
  bool_AirCondFanReq : Inport  Port=2  OutDataType=fixdt(1, 16)  OutScaling=2^0
  st_ChrgrSt : Inport  Port=3  OutDataType=fixdt(1, 16)  OutScaling=2^0
  degC_ChrgrTemp : Inport  Port=4  OutDataType=fixdt(1, 16)  OutScaling=2^0
  degC_DCDCActTemp : Inport  Port=5  OutDataType=fixdt(1, 16)  OutScaling=2^0
  st_MCU1CoolgReq : Inport  Port=6  OutDataType=fixdt(1, 16)  OutScaling=2^0
  st_MCU2CoolgReq : Inport  Port=7  OutDataType=fixdt(1, 16)  OutScaling=2^0
  bool_MotCoolgTaskFlg : Inport  Port=8  OutDataType=fixdt(1, 16)  OutScaling=2^0
  CoolingFanControl : Subsystem
  CoolingPmpControl : Subsystem
  ValveControl : Subsystem
  bool_HiSpdFanCmd : Outport  OutDataType=fixdt(1, 16)  OutScaling=2^0
  bool_LoSpdFanCmd : Outport  Port=2  OutDataType=fixdt(1, 16)  OutScaling=2^0
  pct_Mot1WtrPmpCmd : Outport  Port=3  OutDataType=fixdt(1, 16)  OutScaling=2^0
  pct_Mot2WtrPmpCmd : Outport  Port=4  OutDataType=fixdt(1, 16)  OutScaling=2^0
  bool_RMotorValve2CtrlB : Outport  Port=5
  bool_RMotorValve2CtrlC : Outport  Port=6
  bool_ChargerValve1CtrlB : Outport  Port=7
  bool_ChargerValve1CtrlC : Outport  Port=8
  wires:
  CoolingFanControl/2(bool_LoSpdFanCmd) -> bool_LoSpdFanCmd/1
  CoolingFanControl/1(bool_HiSpdFanCmd) -> bool_HiSpdFanCmd/1
  bool_AirCondFanReq/1 -> CoolingFanControl/2(bool_AirCondFanReq)
  degC_MotCoolgLoopWaterTemp/1 -> CoolingFanControl/1(degC_MotCoolgLoopWaterTemp)
  CoolingPmpControl/1(pct_Mot1WtrPmpCmd) -> pct_Mot1WtrPmpCmd/1
  CoolingPmpControl/2(pct_Mot2WtrPmpCmd) -> pct_Mot2WtrPmpCmd/1
  st_MCU2CoolgReq/1 -> CoolingPmpControl/5(st_MCU2CoolgReq), ValveControl/1(st_MCU2CoolgReq)
  st_MCU1CoolgReq/1 -> CoolingPmpControl/4(st_MCU1CoolgReq)
  degC_DCDCActTemp/1 -> CoolingPmpControl/3(degC_DCDCActTemp)
  degC_ChrgrTemp/1 -> CoolingPmpControl/2(degC_ChrgrTemp), ValveControl/3(degC_ChrgrTemp)
  st_ChrgrSt/1 -> CoolingPmpControl/1(st_ChrgrSt), ValveControl/2(st_ChrgrSt)
  ValveControl/2(bool_RMotorValve2CtrlC) -> bool_RMotorValve2CtrlC/1
  ValveControl/1(bool_RMotorValve2CtrlB) -> bool_RMotorValve2CtrlB/1
  ValveControl/3(bool_ChargerValve1CtrlB) -> bool_ChargerValve1CtrlB/1
  ValveControl/4(bool_ChargerValve1CtrlC) -> bool_ChargerValve1CtrlC/1
  bool_MotCoolgTaskFlg/1 -> CoolingFanControl/3(bool_MotCoolgTaskFlg), CoolingPmpControl/6(bool_MotCoolgTaskFlg), ValveControl/4(bool_MotCoolgTaskFlg)

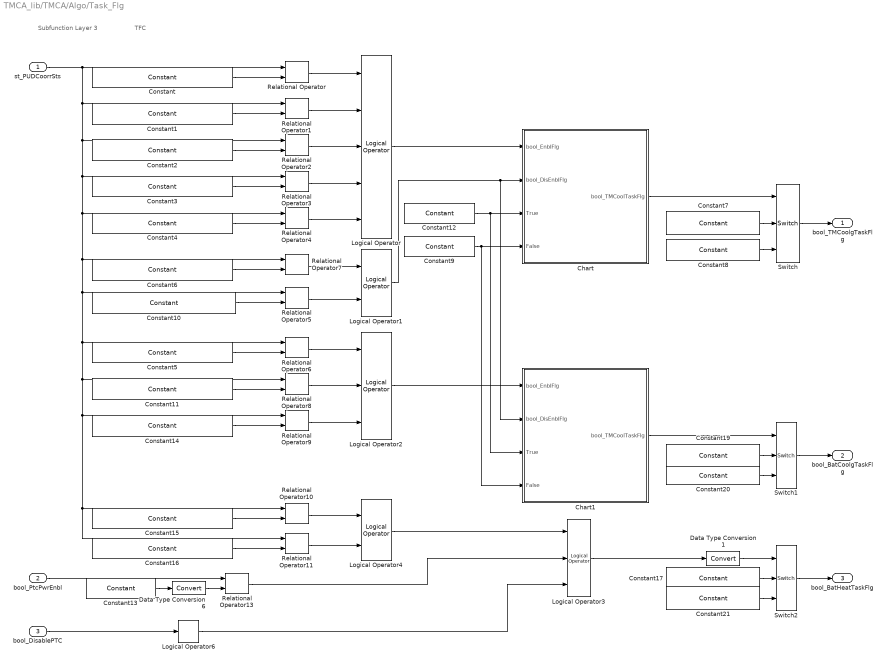
== system TMCA_lib/TMCA/Algo/Task_Flg ==
  note: TFC
  note: Subfunction Layer 3
  st_PUDCoorrSts : Inport
  bool_PtcPwrEnbl : Inport  Port=2
  bool_DisablePTC : Inport  Port=3
  Chart : Stateflow chart  TreatAsAtomicUnit=on
  Chart1 : Stateflow chart  TreatAsAtomicUnit=on
  Constant : BaseOperationLib_Browser/Sources&Sinks/Constant  Value=uint8(PUDCoorrStsTyp.PUD_DrvOn)  OutMin=[]  OutMax=[]  OutDataType=Enum: EgyCoorrStsTyp  ConRadixGroup=Best Precision: Vector-wise  OutScaling=[]  OutDataTypeStr=Inherit: Inherit from 'Constant value'
  Constant1 : BaseOperationLib_Browser/Sources&Sinks/Constant  Value=uint8(PUDCoorrStsTyp.PUD_ACChrgOn)  OutMin=[]  OutMax=[]  OutDataType=Enum: EgyCoorrStsTyp  ConRadixGroup=Best Precision: Vector-wise  OutScaling=[]  OutDataTypeStr=Inherit: Inherit from 'Constant value'
  Constant10 : BaseOperationLib_Browser/Sources&Sinks/Constant  Value=uint8(PUDCoorrStsTyp.PUD_EmgHVOFF_OK)  OutMin=[]  OutMax=[]  OutDataType=Enum: PtCoorrStsTyp  ConRadixGroup=Best Precision: Vector-wise  OutScaling=[]  OutDataTypeStr=Inherit: Inherit from 'Constant value'
  Constant11 : BaseOperationLib_Browser/Sources&Sinks/Constant  Value=uint8(PUDCoorrStsTyp.PUD_ACChrgOn)  OutMin=[]  OutMax=[]  OutDataType=Enum: EgyCoorrStsTyp  ConRadixGroup=Best Precision: Vector-wise  OutScaling=[]  OutDataTypeStr=Inherit: Inherit from 'Constant value'
  Constant12 : BaseOperationLib_Browser/Sources&Sinks/Constant  Value=p_bool_True_M  OutMin=[]  OutMax=[]  OutDataType=fixdt(1, 16)  ConRadixGroup=Use specified scaling  OutScaling=2^0  OutDataTypeStr=Inherit: Inherit from 'Constant value'
  Constant13 : BaseOperationLib_Browser/Sources&Sinks/Constant  Value=p_bool_True_M  OutMin=[]  OutMax=[]  OutDataType=fixdt(1, 16)  ConRadixGroup=Use specified scaling  OutScaling=2^0  OutDataTypeStr=Inherit: Inherit from 'Constant value'
  Constant14 : BaseOperationLib_Browser/Sources&Sinks/Constant  Value=uint8(PUDCoorrStsTyp.PUD_DCChrgOn)  OutMin=[]  OutMax=[]  OutDataType=Enum: EgyCoorrStsTyp  ConRadixGroup=Best Precision: Vector-wise  OutScaling=[]  OutDataTypeStr=Inherit: Inherit from 'Constant value'
  Constant15 : BaseOperationLib_Browser/Sources&Sinks/Constant  Value=uint8(PUDCoorrStsTyp.PUD_ACHeatOn)  OutMin=[]  OutMax=[]  OutDataType=Enum: EgyCoorrStsTyp  ConRadixGroup=Best Precision: Vector-wise  OutScaling=[]  OutDataTypeStr=Inherit: Inherit from 'Constant value'
  Constant16 : BaseOperationLib_Browser/Sources&Sinks/Constant  Value=uint8(PUDCoorrStsTyp.PUD_DCHeatOn)  OutMin=[]  OutMax=[]  OutDataType=Enum: EgyCoorrStsTyp  ConRadixGroup=Best Precision: Vector-wise  OutScaling=[]  OutDataTypeStr=Inherit: Inherit from 'Constant value'
  Constant17 : BaseOperationLib_Browser/Sources&Sinks/Constant  Value=pTMCA_bool_BatHeatEnbl_C  OutMin=[]  OutMax=[]  OutDataType=fixdt(1, 16)  ConRadixGroup=Use specified scaling  OutScaling=2^0  OutDataTypeStr=Inherit: Inherit from 'Constant value'
  Constant19 : BaseOperationLib_Browser/Sources&Sinks/Constant  Value=pTMCA_bool_BatCoolEnbl_C  OutMin=[]  OutMax=[]  OutDataType=fixdt(1, 16)  ConRadixGroup=Use specified scaling  OutScaling=2^0  OutDataTypeStr=Inherit: Inherit from 'Constant value'
  Constant2 : BaseOperationLib_Browser/Sources&Sinks/Constant  Value=uint8(PUDCoorrStsTyp.PUD_DCChrgOn)  OutMin=[]  OutMax=[]  OutDataType=Enum: EgyCoorrStsTyp  ConRadixGroup=Best Precision: Vector-wise  OutScaling=[]  OutDataTypeStr=Inherit: Inherit from 'Constant value'
  Constant{8..9,20..21} (4 alike) : BaseOperationLib_Browser/Sources&Sinks/Constant  Value=p_bool_False_M  OutMin=[]  OutMax=[]  OutDataType=fixdt(1, 16)  ConRadixGroup=Use specified scaling  OutScaling=2^0  OutDataTypeStr=Inherit: Inherit from 'Constant value'
  Constant3 : BaseOperationLib_Browser/Sources&Sinks/Constant  Value=uint8(PUDCoorrStsTyp.PUD_ACHeatOn)  OutMin=[]  OutMax=[]  OutDataType=Enum: EgyCoorrStsTyp  ConRadixGroup=Best Precision: Vector-wise  OutScaling=[]  OutDataTypeStr=Inherit: Inherit from 'Constant value'
  Constant4 : BaseOperationLib_Browser/Sources&Sinks/Constant  Value=uint8(PUDCoorrStsTyp.PUD_DCHeatOn)  OutMin=[]  OutMax=[]  OutDataType=Enum: EgyCoorrStsTyp  ConRadixGroup=Best Precision: Vector-wise  OutScaling=[]  OutDataTypeStr=Inherit: Inherit from 'Constant value'
  Constant5 : BaseOperationLib_Browser/Sources&Sinks/Constant  Value=uint8(PUDCoorrStsTyp.PUD_DrvOn)  OutMin=[]  OutMax=[]  OutDataType=Enum: EgyCoorrStsTyp  ConRadixGroup=Best Precision: Vector-wise  OutScaling=[]  OutDataTypeStr=Inherit: Inherit from 'Constant value'
  Constant6 : BaseOperationLib_Browser/Sources&Sinks/Constant  Value=uint8(PUDCoorrStsTyp.PUD_HVOFF_OK)  OutMin=[]  OutMax=[]  OutDataType=Enum: PtCoorrStsTyp  ConRadixGroup=Best Precision: Vector-wise  OutScaling=[]  OutDataTypeStr=Inherit: Inherit from 'Constant value'
  Constant7 : BaseOperationLib_Browser/Sources&Sinks/Constant  Value=pTMCA_bool_TMCoolEnbl_C  OutMin=[]  OutMax=[]  OutDataType=fixdt(1, 16)  ConRadixGroup=Use specified scaling  OutScaling=2^0  OutDataTypeStr=Inherit: Inherit from 'Constant value'
  Data Type Conversion1 : DataTypeConversion  OutDataType=fixdt(1, 16)  OutScaling=2^0
  Data Type Conversion6 : DataTypeConversion  OutDataType=fixdt(1, 16)  OutScaling=2^0
  Logical Operator : BaseOperationLib_Browser/Logic Operations Changed/Logical Operator  Operator=OR  Inputs=5  AllPortsSameDT=on  OutDataTypeMode=Specify via dialog  LogicDataType=PDT_Bool  OutDataTypeStr=PDT_Bool
  Logical Operator1 : BaseOperationLib_Browser/Logic Operations Changed/Logical Operator  Operator=OR  Inputs=2  AllPortsSameDT=on  OutDataTypeMode=Specify via dialog  LogicDataType=PDT_Bool  OutDataTypeStr=PDT_Bool
  Logical Operator2 : BaseOperationLib_Browser/Logic Operations Changed/Logical Operator  Operator=OR  Inputs=3  AllPortsSameDT=on  OutDataTypeMode=Specify via dialog  LogicDataType=PDT_Bool  OutDataTypeStr=PDT_Bool
  Logical Operator3 : BaseOperationLib_Browser/Logic Operations Changed/Logical Operator  Operator=AND  Inputs=3  AllPortsSameDT=on  OutDataTypeMode=Specify via dialog  LogicDataType=PDT_Bool  OutDataTypeStr=PDT_Bool
  Logical Operator4 : BaseOperationLib_Browser/Logic Operations Changed/Logical Operator  Operator=OR  Inputs=2  AllPortsSameDT=on  OutDataTypeMode=Specify via dialog  LogicDataType=PDT_Bool  OutDataTypeStr=PDT_Bool
  Logical Operator6 : BaseOperationLib_Browser/Logic Operations Changed/Logical Operator  Operator=NOT  Inputs=2  AllPortsSameDT=on  OutDataTypeMode=Specify via dialog  LogicDataType=PDT_Bool  OutDataTypeStr=PDT_Bool
  Relational Operator{,1..11,13} (13 alike) : BaseOperationLib_Browser/Logic Operations Changed/Relational Operator  Operator===  InputSameDT=on  LogicOutDataTypeMode=Specify via dialog  LogicDataType=PDT_Bool  OutDataTypeStr=PDT_Bool
  Switch : BaseOperationLib_Browser/Signal Routing Changed/Switch  Criteria=u2 ~= 0  Threshold=1  InputSameDT=on  OutMin=[]  OutMax=[]  OutDataType=fixdt(1,16,0)  OutScaling=[]  SaturateOnIntegerOverflow=on
  Switch1 : BaseOperationLib_Browser/Signal Routing Changed/Switch  Criteria=u2 ~= 0  Threshold=1  InputSameDT=on  OutMin=[]  OutMax=[]  OutDataType=fixdt(1,16,0)  OutScaling=[]  SaturateOnIntegerOverflow=on
  Switch2 : BaseOperationLib_Browser/Signal Routing Changed/Switch  Criteria=u2 ~= 0  Threshold=1  InputSameDT=on  OutMin=[]  OutMax=[]  OutDataType=fixdt(1,16,0)  OutScaling=[]  SaturateOnIntegerOverflow=on
  bool_TMCoolgTaskFlg : Outport  OutDataType=fixdt(1, 16)  OutScaling=2^0
  bool_BatCoolgTaskFlg : Outport  Port=2  OutDataType=fixdt(1, 16)  OutScaling=2^0
  bool_BatHeatTaskFlg : Outport  Port=3  OutDataType=fixdt(1, 16)  OutScaling=2^0
  wires:
  Constant1/1 -> Relational Operator1/2
  Constant2/1 -> Relational Operator2/2
  Constant3/1 -> Relational Operator3/2
  Relational Operator/1 -> Logical Operator/1
  Relational Operator1/1 -> Logical Operator/2
  Relational Operator2/1 -> Logical Operator/3
  Relational Operator3/1 -> Logical Operator/4
  Relational Operator4/1 -> Logical Operator/5
  st_PUDCoorrSts/1 -> Relational Operator/1, Relational Operator1/1, Relational Operator2/1, Relational Operator3/1, Relational Operator4/1, Relational Operator7/1, Relational Operator8/1, Relational Operator9/1, Relational Operator10/1, Relational Operator11/1, Relational Operator6/1, Relational Operator5/1
  Logical Operator/1 -> Chart/1(bool_EnblFlg)
  Constant9/1 -> Chart1/4(False), Chart/4(False)
  Constant12/1 -> Chart1/3(True), Chart/3(True)
  Constant6/1 -> Relational Operator7/2
  Logical Operator1/1 -> Chart1/2(bool_DisEnblFlg), Chart/2(bool_DisEnblFlg)
  Switch/1 -> bool_TMCoolgTaskFlg/1
  Constant7/1 -> Switch/2
  Chart/1(bool_TMCoolTaskFlg) -> Switch/1
  Constant10/1 -> Relational Operator5/2
  Relational Operator7/1 -> Logical Operator1/1
  Relational Operator5/1 -> Logical Operator1/2
  Constant/1 -> Relational Operator/2
  Constant4/1 -> Relational Operator4/2
  Constant8/1 -> Switch/3
  Data Type Conversion6/1 -> Relational Operator13/2
  Constant20/1 -> Switch1/3
  Constant19/1 -> Switch1/2
  Switch1/1 -> bool_BatCoolgTaskFlg/1
  Relational Operator11/1 -> Logical Operator4/2
  Relational Operator10/1 -> Logical Operator4/1
  Relational Operator9/1 -> Logical Operator2/3
  Relational Operator8/1 -> Logical Operator2/2
  Relational Operator6/1 -> Logical Operator2/1
  Constant16/1 -> Relational Operator11/2
  Constant15/1 -> Relational Operator10/2
  Constant14/1 -> Relational Operator9/2
  Constant11/1 -> Relational Operator8/2
  Constant5/1 -> Relational Operator6/2
  Constant17/1 -> Switch2/2
  Logical Operator4/1 -> Logical Operator3/1
  Switch2/1 -> bool_BatHeatTaskFlg/1
  Logical Operator3/1 -> Data Type Conversion1/1
  Constant21/1 -> Switch2/3
  bool_PtcPwrEnbl/1 -> Relational Operator13/1
  Constant13/1 -> Data Type Conversion6/1
  Relational Operator13/1 -> Logical Operator3/2
  Data Type Conversion1/1 -> Switch2/1
  Chart1/1(bool_TMCoolTaskFlg) -> Switch1/1
  bool_DisablePTC/1 -> Logical Operator6/1
  Logical Operator6/1 -> Logical Operator3/3
  Logical Operator2/1 -> Chart1/1(bool_EnblFlg)

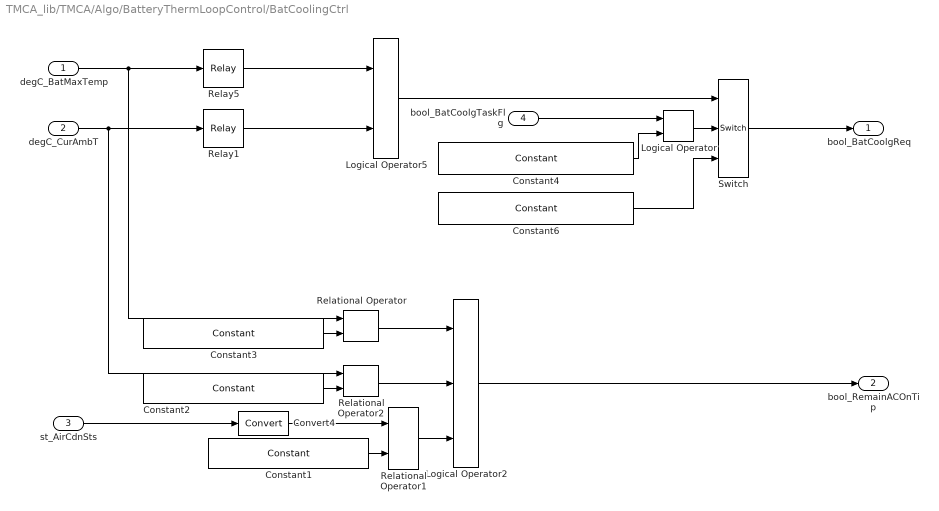
== system TMCA_lib/TMCA/Algo/BatteryThermLoopControl/BatCoolingCtrl ==
  degC_BatMaxTemp : Inport  OutDataType=fixdt(1, 16)  OutScaling=2^0
  degC_CurAmbT : Inport  Port=2  OutDataType=fixdt(1, 16)  OutScaling=2^0
  st_AirCdnSts : Inport  Port=3  OutDataType=fixdt(1, 16)  OutScaling=2^0
  bool_BatCoolgTaskFlg : Inport  Port=4  OutDataType=fixdt(1, 16)  OutScaling=2^0
  Constant1 : BaseOperationLib_Browser/Sources&Sinks/Constant  Value=pTMCA_st_AirCdnOn_C  OutMin=[]  OutMax=[]  OutDataType=fixdt(1, 16)  ConRadixGroup=Use specified scaling  OutScaling=2^0  OutDataTypeStr=Inherit: Inherit from 'Constant value'
  Constant2 : BaseOperationLib_Browser/Sources&Sinks/Constant  Value=pTMCA_degC_AmbHiTempDisply_C  OutMin=[]  OutMax=[]  OutDataType=fixdt(1, 16)  ConRadixGroup=Use specified scaling  OutScaling=2^0  OutDataTypeStr=Inherit: Inherit from 'Constant value'
  Constant3 : BaseOperationLib_Browser/Sources&Sinks/Constant  Value=pTMCA_degC_BatHiTempDisply_C  OutMin=[]  OutMax=[]  OutDataType=fixdt(1, 16)  ConRadixGroup=Use specified scaling  OutScaling=2^0  OutDataTypeStr=Inherit: Inherit from 'Constant value'
  Constant4 : BaseOperationLib_Browser/Sources&Sinks/Constant  Value=pTMCA_bool_BatCoolACReqEnbl_C  OutMin=[]  OutMax=[]  OutDataType=fixdt(1, 16)  ConRadixGroup=Use specified scaling  OutScaling=2^0  OutDataTypeStr=Inherit: Inherit from 'Constant value'
  Constant6 : BaseOperationLib_Browser/Sources&Sinks/Constant  Value=pTMCA_bool_BatCoolACReqCtrl_C  OutMin=[]  OutMax=[]  OutDataType=fixdt(1, 16)  ConRadixGroup=Use specified scaling  OutScaling=2^0  OutDataTypeStr=Inherit: Inherit from 'Constant value'
  Convert4 : DataTypeConversion  OutDataType=fixdt(1, 16)  OutScaling=2^0
  Logical Operator : BaseOperationLib_Browser/Logic Operations Changed/Logical Operator  Operator=AND  Inputs=2  AllPortsSameDT=on  OutDataTypeMode=Specify via dialog  LogicDataType=PDT_Bool  OutDataTypeStr=PDT_Bool
  Logical Operator2 : BaseOperationLib_Browser/Logic Operations Changed/Logical Operator  Operator=AND  Inputs=3  AllPortsSameDT=on  OutDataTypeMode=Specify via dialog  LogicDataType=PDT_Bool  OutDataTypeStr=PDT_Bool
  Logical Operator5 : BaseOperationLib_Browser/Logic Operations Changed/Logical Operator  Operator=AND  Inputs=2  AllPortsSameDT=on  OutDataTypeMode=Specify via dialog  LogicDataType=PDT_Bool  OutDataTypeStr=PDT_Bool
  Relational Operator : BaseOperationLib_Browser/Logic Operations Changed/Relational Operator  Operator=<=  InputSameDT=on  LogicOutDataTypeMode=Specify via dialog  LogicDataType=PDT_Bool  OutDataTypeStr=PDT_Bool
  Relational Operator1 : BaseOperationLib_Browser/Logic Operations Changed/Relational Operator  Operator===  InputSameDT=on  LogicOutDataTypeMode=Specify via dialog  LogicDataType=PDT_Bool  OutDataTypeStr=PDT_Bool
  Relational Operator2 : BaseOperationLib_Browser/Logic Operations Changed/Relational Operator  Operator=<=  InputSameDT=on  LogicOutDataTypeMode=Specify via dialog  LogicDataType=PDT_Bool  OutDataTypeStr=PDT_Bool
  Relay1 : BaseOperationLib_Browser/Discontinuities Changed/Relay  OnSwitchValue=pTMCA_degC_BatCoolAmbHiTemp_C  OffSwitchValue=pTMCA_degC_BatCoolAmbLoTemp_C  OnOutputValue=p_bool_True_M  OffOutputValue=p_bool_False_M  OutMin=[]  OutMax=[]  OutDataType=fixdt(1, 16)  ConRadixGroup=Use specified scaling  OutScaling=2^0  OutDataTypeStr=Inherit: Inherit via back propagation
      settings: AttributesFormatString=%<OnSwitchValue> OnOut %<OnOutputValue>\n%<OffSwitchValue> OffOut %<OffOutputValue>
  Relay5 : BaseOperationLib_Browser/Discontinuities Changed/Relay  OnSwitchValue=pTMCA_degC_BatCoolHiTemp_C  OffSwitchValue=pTMCA_degC_BatCoolLoTemp_C  OnOutputValue=p_bool_True_M  OffOutputValue=p_bool_False_M  OutMin=[]  OutMax=[]  OutDataType=fixdt(1, 16)  ConRadixGroup=Use specified scaling  OutScaling=2^0  OutDataTypeStr=Inherit: Inherit via back propagation
      settings: AttributesFormatString=%<OnSwitchValue> OnOut %<OnOutputValue>\n%<OffSwitchValue> OffOut %<OffOutputValue>
  Switch : BaseOperationLib_Browser/Signal Routing Changed/Switch  Criteria=u2 ~= 0  Threshold=1  InputSameDT=on  OutMin=[]  OutMax=[]  OutDataType=fixdt(1,16,0)  OutScaling=[]  SaturateOnIntegerOverflow=on
  bool_BatCoolgReq : Outport  OutDataType=fixdt(1, 16)  OutScaling=2^0
  bool_RemainACOnTip : Outport  Port=2  OutDataType=fixdt(1, 16)  OutScaling=2^0
  wires:
  Constant3/1 -> Relational Operator/2
  Constant2/1 -> Relational Operator2/2
  Relational Operator2/1 -> Logical Operator2/2
  Relational Operator/1 -> Logical Operator2/1
  Relational Operator1/1 -> Logical Operator2/3
  degC_CurAmbT/1 -> Relational Operator2/1, Relay1/1
  Relay1/1 -> Logical Operator5/2
  bool_BatCoolgTaskFlg/1 -> Logical Operator/1
  Constant4/1 -> Logical Operator/2
  Logical Operator/1 -> Switch/2
  Convert4/1 -> Relational Operator1/1
  Logical Operator2/1 -> bool_RemainACOnTip/1
  Logical Operator5/1 -> Switch/1
  st_AirCdnSts/1 -> Convert4/1
  Constant1/1 -> Relational Operator1/2
  degC_BatMaxTemp/1 -> Relational Operator/1, Relay5/1
  Relay5/1 -> Logical Operator5/1
  Constant6/1 -> Switch/3
  Switch/1 -> bool_BatCoolgReq/1

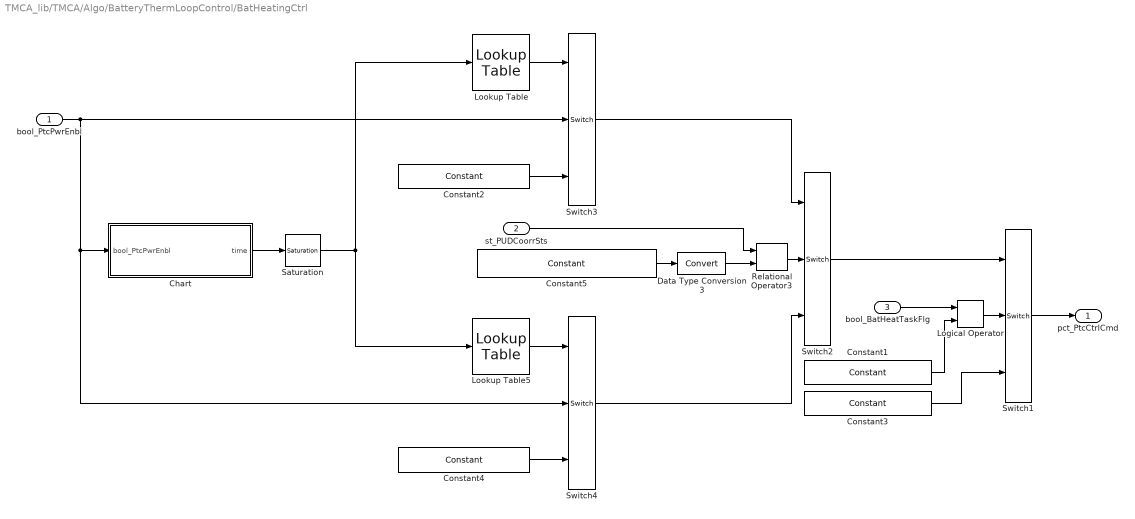
== system TMCA_lib/TMCA/Algo/BatteryThermLoopControl/BatHeatingCtrl ==
  bool_PtcPwrEnbl : Inport  OutDataType=fixdt(1, 16)  OutScaling=2^0
  st_PUDCoorrSts : Inport  Port=2  OutDataType=fixdt(1, 16)  OutScaling=2^0
  bool_BatHeatTaskFlg : Inport  Port=3  OutDataType=fixdt(1, 16)  OutScaling=2^0
  Chart : Stateflow chart  TreatAsAtomicUnit=on
  Constant1 : BaseOperationLib_Browser/Sources&Sinks/Constant  Value=pTMCA_pct_HeatPTCEnbl_C  OutMin=[]  OutMax=[]  OutDataType=fixdt(1, 16)  ConRadixGroup=Use specified scaling  OutScaling=2^0  OutDataTypeStr=Inherit: Inherit from 'Constant value'
  Constant2 : BaseOperationLib_Browser/Sources&Sinks/Constant  Value=pTMCA_pct_HeatrOffVal_C  OutMin=[]  OutMax=[]  OutDataType=fixdt(1, 16)  ConRadixGroup=Use specified scaling  OutScaling=2^0  OutDataTypeStr=Inherit: Inherit from 'Constant value'
  Constant3 : BaseOperationLib_Browser/Sources&Sinks/Constant  Value=pTMCA_pct_HeatPTCCtrl_C  OutMin=[]  OutMax=[]  OutDataType=fixdt(1, 16)  ConRadixGroup=Use specified scaling  OutScaling=2^0  OutDataTypeStr=Inherit: Inherit from 'Constant value'
  Constant4 : BaseOperationLib_Browser/Sources&Sinks/Constant  Value=pTMCA_pct_HeatrOffVal_C  OutMin=[]  OutMax=[]  OutDataType=fixdt(1, 16)  ConRadixGroup=Use specified scaling  OutScaling=2^0  OutDataTypeStr=Inherit: Inherit from 'Constant value'
  Constant5 : BaseOperationLib_Browser/Sources&Sinks/Constant  Value=uint8(PUDCoorrStsTyp.PUD_ACHeatOn)  OutMin=[]  OutMax=[]  OutDataType=Enum: EgyCoorrStsTyp  ConRadixGroup=Best Precision: Vector-wise  OutScaling=[]  OutDataTypeStr=Inherit: Inherit from 'Constant value'
  Data Type Conversion3 : DataTypeConversion  OutDataType=fixdt(1, 16)  OutScaling=2^0
  Logical Operator : BaseOperationLib_Browser/Logic Operations Changed/Logical Operator  Operator=AND  Inputs=2  AllPortsSameDT=on  OutDataTypeMode=Specify via dialog  LogicDataType=PDT_Bool  OutDataTypeStr=PDT_Bool
  Lookup Table : BaseOperationLib_Browser/Lookup Tables Changed/Lookup Table  InputValues=pTMCA_cnt_ACHeatTime_CUR  Table=pTMCA_pct_ACHeatPTCPWM_CUR  LookUpMeth=Interpolation-Use End Values  OutMin=[]  OutMax=[]  OutDataType=fixdt(1, 16)  OutScaling=2^0  OutDataTypeStr=Inherit: Inherit via back propagation  SaturateOnIntegerOverflow=on
      settings: AttributesFormatString=X:%<InputValues>\nTAB:%<Table>
  Lookup Table5 : BaseOperationLib_Browser/Lookup Tables Changed/Lookup Table  InputValues=pTMCA_cnt_DCTempTime_CUR  Table=pTMCA_pct_DCHeatPTCPWM_CUR  LookUpMeth=Interpolation-Use End Values  OutMin=[]  OutMax=[]  OutDataType=fixdt(1, 16)  OutScaling=2^0  OutDataTypeStr=Inherit: Inherit via back propagation  SaturateOnIntegerOverflow=on
      settings: AttributesFormatString=X:%<InputValues>\nTAB:%<Table>
  Relational Operator3 : BaseOperationLib_Browser/Logic Operations Changed/Relational Operator  Operator===  InputSameDT=on  LogicOutDataTypeMode=Specify via dialog  LogicDataType=PDT_Bool  OutDataTypeStr=PDT_Bool
  Saturation : BaseOperationLib_Browser/Discontinuities Unchanged/Saturation  UpperLimit=pTMCA_cnt_TimeUpLim_C  LowerLimit=pTMCA_cnt_TimeDwnLim_C  OutMin=[]  OutMax=[]  OutDataType=fixdt(1, 16)  OutScaling=2^0
      settings: AttributesFormatString=ULim:%<UpperLimit>\nLLim:%<LowerLimit>
  Switch{1..4} (4 alike) : BaseOperationLib_Browser/Signal Routing Changed/Switch  Criteria=u2 ~= 0  Threshold=1  InputSameDT=on  OutMin=[]  OutMax=[]  OutDataType=fixdt(1,16,0)  OutScaling=[]  SaturateOnIntegerOverflow=on
  pct_PtcCtrlCmd : Outport  OutDataType=fixdt(1, 16)  OutScaling=2^0
  wires:
  Saturation/1 -> Lookup Table5/1, Lookup Table/1
  Lookup Table/1 -> Switch3/1
  Lookup Table5/1 -> Switch4/1
  Chart/1(time) -> Saturation/1
  Constant4/1 -> Switch4/3
  Constant2/1 -> Switch3/3
  bool_PtcPwrEnbl/1 -> Chart/1(bool_PtcPwrEnbl), Switch4/2, Switch3/2
  Switch1/1 -> pct_PtcCtrlCmd/1
  Data Type Conversion3/1 -> Relational Operator3/2
  Constant5/1 -> Data Type Conversion3/1
  st_PUDCoorrSts/1 -> Relational Operator3/1
  Relational Operator3/1 -> Switch2/2
  Switch3/1 -> Switch2/1
  Switch4/1 -> Switch2/3
  Switch2/1 -> Switch1/1
  Logical Operator/1 -> Switch1/2
  bool_BatHeatTaskFlg/1 -> Logical Operator/1
  Constant1/1 -> Logical Operator/2
  Constant3/1 -> Switch1/3
